simulink model "Cruise_Control_PI_Control"  (R2017b)
settings: Solver=VariableStepAuto  StartTime=0.0  StopTime=10.0  RelTol=1e-3
InitFcn:
  | InitCruiseControl
values from neighbouring files (symbols this model uses):
  b = 10    [InitCruiseControl.m]
  Ki = 0    [InitCruiseControl.m]
  Kp = 5.46    [InitCruiseControl.m]
  m = 1000    [InitCruiseControl.m]
settings Model: Creator=rizwanahmed  LastModifiedBy=rizwanahmed

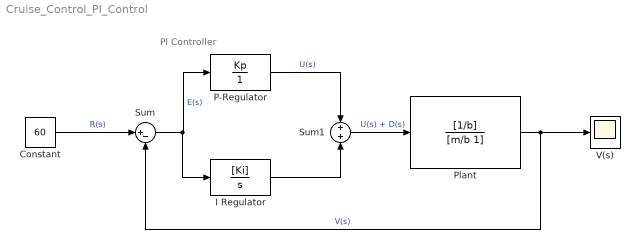
== system Cruise_Control_PI_Control ==
  note: PI Controller
  " Plant" : TransferFcn  Numerator=[1/b]  Denominator=[m/b 1]
  Constant : Constant  Value=60
  I Regulator : TransferFcn  Numerator=[Ki]  Denominator=[1 0]
  P-Regulator : TransferFcn  Numerator=Kp  Denominator=[0 1]
  Sum : Sum  Inputs=|+-
  Sum1 : Sum
  V(s) : Scope
  wires:
  Constant/1 -> Sum/1  "R(s)"
  Sum/1 -> I Regulator/1, P-Regulator/1  "E(s)"
  " Plant"/1 -> Sum/2, V(s)/1  "V(s)"
  Sum1/1 -> " Plant"/1  "U(s) + D(s)"
  P-Regulator/1 -> Sum1/1  "U(s)"
  I Regulator/1 -> Sum1/2
